simulink model "SIGMA"  (Simulink 6.0)
settings: Solver=VariableStepDiscrete  StartTime=0.0  StopTime=100  MaxStep=0.05  RelTol=1e-3
libraries: simulink x3
settings Model: LastModifiedBy=root

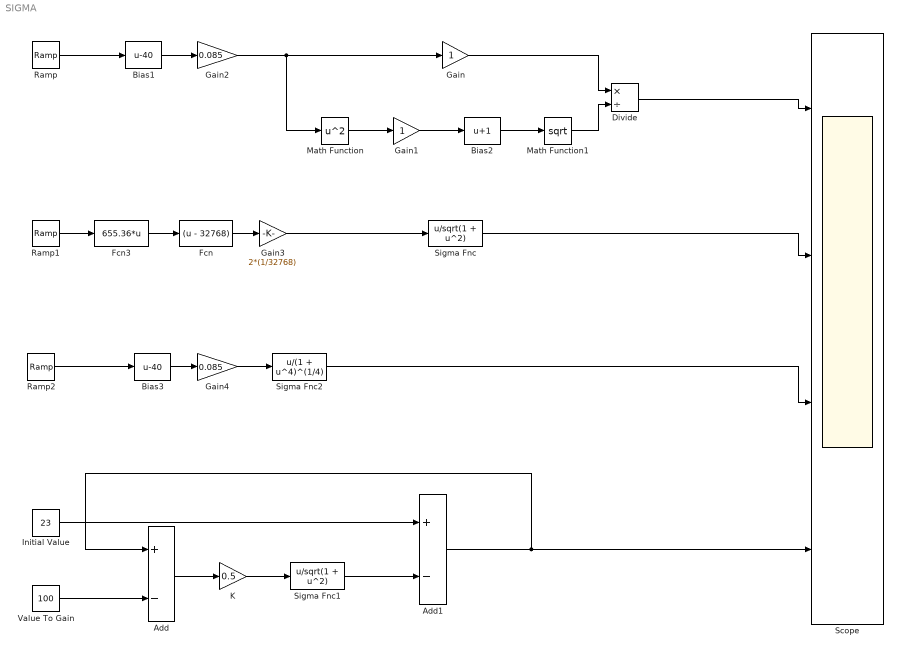
== system SIGMA ==
  Add : Sum  Inputs=+-  OutScaling=2^-10
  Add1 : Sum  Inputs=+-  OutScaling=2^-10
  Bias1 : Bias  Bias=-40
  Bias2 : Bias  Bias=1
  Bias3 : Bias  Bias=-40
  Divide : Product  Inputs=*/  OutScaling=2^-10
  Fcn : Fcn  Expr=(u - 32768)
  Fcn3 : Fcn  Expr=655.36*u
  Gain : Gain
  Gain1 : Gain
  Gain2 : Gain  Gain=0.085
  Gain3 : Gain  Gain=2*(1/32768)
  Gain4 : Gain  Gain=0.085
  Initial Value : Constant  Value=23
  K : Gain  Gain=0.5
  Math Function : Math  Operator=square  SaturateOnIntegerOverflow=on
  Math Function1 : Math  Operator=sqrt  SaturateOnIntegerOverflow=on
  Ramp : simulink/Sources/Ramp  slope=1  start=0  X0=0
  Ramp1 : simulink/Sources/Ramp  slope=1  start=0  X0=0
  Ramp2 : simulink/Sources/Ramp  slope=1  start=0  X0=0
  Scope : Scope  NumInputPorts=4
      settings: TickLabels=on  TimeRange=100  YMin=-1.5~-1.5~-1~0  YMax=1.5~1.5~1~100
  Sigma Fnc : Fcn  Expr=u/sqrt(1 + u^2)
  Sigma Fnc1 : Fcn  Expr=u/sqrt(1 + u^2)
  Sigma Fnc2 : Fcn  Expr=u/(1 + u^4)^(1/4)
  Value To Gain : Constant  Value=100
  wires:
  Gain/1 -> Divide/1
  Math Function/1 -> Gain1/1
  Gain1/1 -> Bias2/1
  Bias2/1 -> Math Function1/1
  Math Function1/1 -> Divide/2
  Divide/1 -> Scope/1
  Bias1/1 -> Gain2/1
  Sigma Fnc/1 -> Scope/2
  Ramp/1 -> Bias1/1
  Fcn/1 -> Gain3/1
  Gain2/1 -> Gain/1, Math Function/1
  Ramp1/1 -> Fcn3/1
  Gain3/1 -> Sigma Fnc/1
  Fcn3/1 -> Fcn/1
  Value To Gain/1 -> Add/2
  Add/1 -> K/1
  K/1 -> Sigma Fnc1/1
  Sigma Fnc1/1 -> Add1/2
  Ramp2/1 -> Bias3/1
  Sigma Fnc2/1 -> Scope/3
  Add1/1 -> Add/1, Scope/4
  Initial Value/1 -> Add1/1
  Bias3/1 -> Gain4/1
  Gain4/1 -> Sigma Fnc2/1
